simulink model "Problem_2"  (R2020a)
settings: Solver=VariableStepAuto  StartTime=0.0  StopTime=10.0  RelTol=1e-3
model workspace (MAT data in the model file):
  K1 = Simulink.Parameter
  K1.Value = 50
  K1.DataType = 'auto'
  K1.Dimensions = [1 1]
  K2 = Simulink.Parameter
  K2.Value = 40
  K2.DataType = 'auto'
  K2.Dimensions = [1 1]
  M1 = Simulink.Parameter
  M1.Value = 100
  M1.DataType = 'auto'
  M1.Dimensions = [1 1]
  M2 = Simulink.Parameter
  M2.Value = 80
  M2.DataType = 'auto'
  M2.Dimensions = [1 1]
  b = Simulink.Parameter
  b.Value = 50
  b.DataType = 'auto'
  b.Dimensions = [1 1]
settings Model: Creator=hp  LastModifiedBy=hp

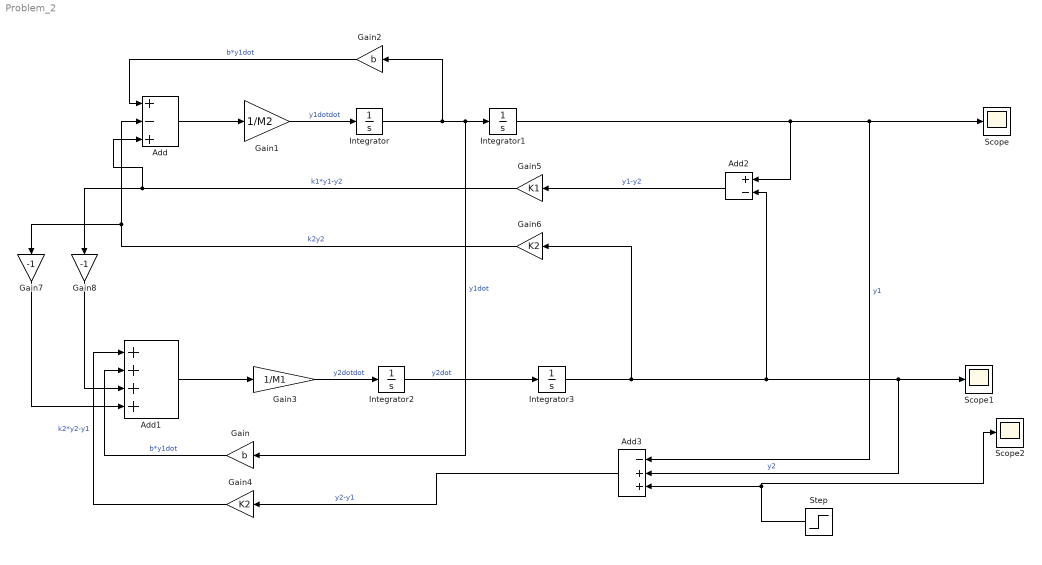
== system Problem_2 ==
  Add : Sum  Inputs=+-+
  Add1 : Sum  Inputs=++++
  Add2 : Sum  Inputs=+-
  Add3 : Sum  Inputs=-++
  Gain : Gain  Gain=b
  Gain1 : Gain  Gain=1/M2
  Gain2 : Gain  Gain=b
  Gain3 : Gain  Gain=1/M1
  Gain4 : Gain  Gain=K2
  Gain5 : Gain  Gain=K1
  Gain6 : Gain  Gain=K2
  Gain7 : Gain  Gain=-1
  Gain8 : Gain  Gain=-1
  Integrator{,1..3} (4 alike) : Integrator
  Scope : Scope
  Scope1 : Scope
  Scope2 : Scope
  Step : Step  SampleTime=0
  wires:
  Add/1 -> Gain1/1
  Gain1/1 -> Integrator/1  "y1dotdot"
  Integrator/1 -> Gain2/1, Gain/1, Integrator1/1  "y1dot"
  Integrator1/1 -> Add2/1, Add3/1, Scope/1  "y1"
  Gain2/1 -> Add/1  "b*y1dot"
  Gain8/1 -> Add1/3
  Gain7/1 -> Add1/4
  Gain/1 -> Add1/2  "b*y1dot"
  Gain4/1 -> Add1/1  "k2*y2-y1"
  Add1/1 -> Gain3/1
  Gain3/1 -> Integrator2/1  "y2dotdot"
  Integrator2/1 -> Integrator3/1  "y2dot"
  Integrator3/1 -> Gain6/1, Add2/2, Add3/2, Scope1/1  "y2"
  Add2/1 -> Gain5/1  "y1-y2"
  Step/1 -> Scope2/1, Add3/3
  Add3/1 -> Gain4/1  "y2-y1"
  Gain5/1 -> Add/3, Gain8/1  "k1*y1-y2"
  Gain6/1 -> Gain7/1, Add/2  "k2y2"
